simulink library "dspobslib"  (Simulink 6.0)
values from neighbouring files (symbols this model uses):
  D = D + B    [rebuffer_delay.m]
libraries: dspsigattribs x15, simulink x10, dspobslib x3, dspbuff3 x2, dspmtrx3 x2, dspmathops x1
settings Model: RequirementInfo=9  CovMetricSettings=d  Creator=don  LastModifiedBy=mlongfri  ExtModeAutoUpdateStatusClock=off  ProdHWDeviceType=Specified

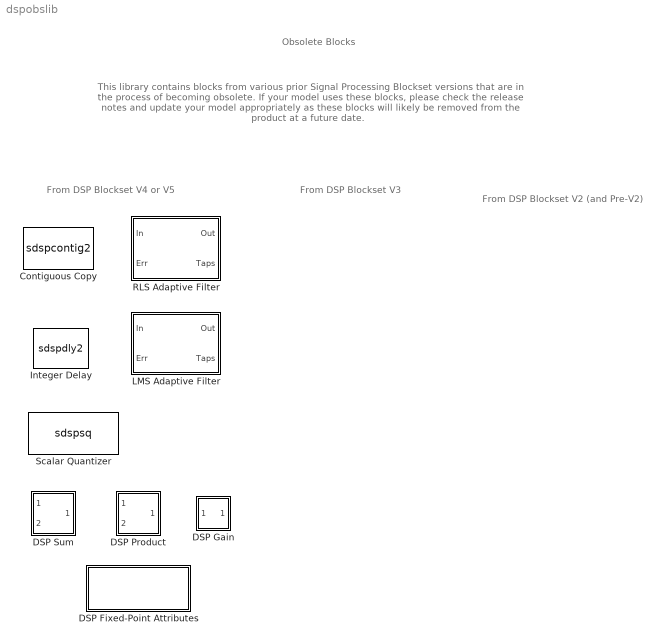
== system dspobslib ==
  note: Obsolete Blocks
  note: This library contains blocks from various prior Signal Processing Blockset versions
      | that are in the process of becoming obsolete. If your model uses these blocks, please
      | check the release notes and update your model appropriately as these blocks will likely
      | be removed from the product at a future date.
  note: From DSP Blockset V4 or V5
  note: From DSP Blockset V3
  note: From DSP Blockset V2
      | (and Pre-V2)
  Contiguous Copy : S-Function  FunctionName=sdspcontig2
      mask Type: Contiguous Copy
      mask Description: Create a contiguous copy of input data.  For use with blocks that only accept contiguous data during simulation or code generation.
      mask Help: web(dspbhelp);
      mask Display: disp('Contiguous\nCopy');
  DSP Fixed-Point Attributes : Subsystem  mask(DSP Fixed-Point Attributes){outputSource=Inherit, outputWordLength=16, outputFracLength=15, accumSource=Inherit, accumWordLength=32, accumFracLength=30, prodOutputSource=Inherit, prodOutputWordLength=32, prodOutputFracLength=30, memorySource=Inherit, memoryWordLength=16, memoryFracLength=15, miscSource=Inherit, roundingMode=Floor, overflowMode=off}
      mask prompts: outputSource "Where from (out)?"; outputWordLength "Word length:"; outputFracLength "Fraction length:"; accumSource "Where from (acc)?"; accumWordLength "Word length:"; accumFracLength "Fraction length:"; prodOutputSource "Where from (po)?"; prodOutputWordLength "Word length:"; prodOutputFracLength "Fraction length:"; memorySource "Where from (mem)?"; memoryWordLength "Word length:"; memoryFracLength "Fraction length:"; miscSource "Where from (misc)?"; roundingMode "Round integer calculations towards:"; overflowMode "Saturate on integer overflow"
      mask help: Sets fixed-point parameters on a model-wide (if at root level) or subsystem-wide basis. Blocks that have 'Inherit from master dialog' will use the parameters specified here unless overridden at a lower level.
      settings: CopyFcn=dspFixptManager('addController');  DeleteFcn=dspFixptManager('removeController');  UndoDeleteFcn=dspFixptManager('addController');  ModelCloseFcn=dspFixptManager('closeModel');  NameChangeFcn=dspFixptManager('changeName');  OpenFcn=dspFixptManager('openUI');
      mask Help: web(dspbhelp);
      mask StyleString: popup(Local|Inherit),edit,edit,popup(Local|Inherit),edit,edit,popup(Local|Inherit),edit,edit,popup(Local|Inherit),edit,edit,popup(Local|Inherit),popup(Floor|Nearest),checkbox
      mask CallbackString: dspblkFPA('out');|||dspblkFPA('acc');|||dspblkFPA('po');|||dspblkFPA('mem');|||dspblkFPA('misc');||
      mask Display: disp('DSP Fixed-Point\nAttributes','horizontalalign','center')
  DSP Gain : Subsystem  mask(DSP Gain){gainValue=1, additionalParams=off, allowOverrides=on, gainMode=Same as input, gainWordLength=16, gainFracLength=15, prodOutputMode=Same as input, prodOutputWordLength=32, prodOutputFracLength=30, roundingMode=Floor, overflowMode=off}
      mask prompts: gainValue "Gain value:"; additionalParams "------- Show additional parameters --------"; allowOverrides "Allow overrides from DSP Fixed-Point Attributes blocks"; gainMode "Fixed-point gain attributes:"; gainWordLength "Gain word length:"; gainFracLength "Gain fraction length:"; prodOutputMode "Fixed-point output attributes:"; prodOutputWordLength "Output word length:"; prodOutputFracLength "Output fraction length:"; roundingMode "Round integer calculations toward:"; overflowMode "Saturate on integer overflow"
      mask help: Apply element-wise gain to input. Any fixed-point settings are ignored for floating-point inputs.
      mask init:
      | iconStr = dspblkdspgain('icon');
      | dspblkdspgain('init');
      mask Help: web(dspbhelp);
      mask StyleString: edit,checkbox,checkbox,popup(Same as input|User-defined),edit,edit,popup(Same as input|User-defined),edit,edit,popup(Floor|Nearest),checkbox
      mask CallbackString: |dspblkdspgain;|dspblkdspgain;|dspblkdspgain;|||dspblkdspgain;|||dspblkdspgain;|dspblkdspgain;
      mask Display:
      | text(0.309,0.5,iconStr,'horizontalalignment','center')
      | plot([0,0],[0,1]);
      | plot([0,1],[0,0.5]);
      | plot([0,1],[1,0.5]);
  DSP Product : Subsystem  mask(DSP Product){allowOverrides=on, prodOutputMode=Same as first input, prodOutputWordLength=32, prodOutputFracLength=30, roundingMode=Floor, overflowMode=off}
      mask prompts: allowOverrides "Allow overrides from DSP Fixed-Point Attributes blocks"; prodOutputMode "Fixed-point output attributes:"; prodOutputWordLength "Output word length:"; prodOutputFracLength "Output fraction length:"; roundingMode "Round integer calculations toward:"; overflowMode "Saturate on integer overflow"
      mask help: Perform element-wise multiplication on two inputs. Any fixed-point settings are ignored for floating-point inputs.
      mask init:
      | dspblksummult('init','Product')
      | dspblksummult('update','Product')
      mask Help: web(dspbhelp);
      mask StyleString: checkbox,popup(Same as first input|User-defined),edit,edit,popup(Floor|Nearest),checkbox
      mask CallbackString: dspblksummult('Product');|dspblksummult('Product');|||dspblksummult('Product');|dspblksummult('Product');
      mask Display:
      | plot((0.5+cos([0:3:360]*pi/180)/3),(0.5+sin([0:3:360]*pi/180)/3))
      | plot([.35,.65],[.35,.65])
      | plot([.65,.35],[.35,.65])
  DSP Sum : Subsystem  mask(DSP Sum){allowOverrides=on, accumMode=Same as first input, accumWordLength=32, accumFracLength=30, roundingMode=Floor, overflowMode=off}
      mask prompts: allowOverrides "Allow overrides from DSP Fixed-Point Attributes blocks"; accumMode "Fixed-point output attributes:"; accumWordLength "Output word length:"; accumFracLength "Output fraction length:"; roundingMode "Round integer calculations toward:"; overflowMode "Saturate on integer overflow"
      mask help: Sum two inputs. Any fixed-point settings are ignored for floating-point inputs.
      mask init:
      | dspblksummult('init','Sum')
      | dspblksummult('update','Sum')
      mask Help: web(dspbhelp);
      mask StyleString: checkbox,popup(Same as first input|User-defined),edit,edit,popup(Floor|Nearest),checkbox
      mask CallbackString: dspblksummult('Sum');|dspblksummult('Sum');|||dspblksummult('Sum');|dspblksummult('Sum');
      mask Display:
      | plot((0.5+cos([0:3:360]*pi/180)/3),(0.5+sin([0:3:360]*pi/180)/3))
      | plot([.5,.5],[.35,.65])
      | plot([.35,.65],[.5,.5])
  Integer Delay : S-Function  FunctionName=sdspdly2  Parameters=delay,ic,reset  mask(Integer Delay){delay=1, ic=0, reset_popup=None}
      mask prompts: delay "Delay (samples):"; ic "Initial conditions:"; reset_popup "Reset port:"
      mask help: Delay discrete-time input by a fixed integer number of sample periods.
      mask init:
      | str = dspblkdly2('icon',&1,delay);
      | dx = 0.01*length(str);
      | reset = reset_popup-1;
      | if (reset == 0)
      | 	s.i1 = 1; s.i1s = '';
      | 	s.i2 = 1; s.i2s = '';
      | else
      | 	s.i1 = 1; s.i1s = 'In';
      | 	s.i2 = 2; s.i2s = 'Rst';
      | end
      mask Help: web(dspbhelp);
      mask StyleString: edit,edit,popup(None|Rising edge|Falling edge|Either edge|Non-zero sample)
      mask Display:
      | text(0.42-dx, 0.4, 'z'); text(0.5-dx, 0.6, str);
      | port_label('input',s.i1,s.i1s);
      | port_label('input',s.i2,s.i2s);
  LMS Adaptive Filter : Subsystem  mask(LMS Adaptive Filter){n=32, mu=.65, ic=0.0, leakage=1.0, normalized=on, Adapt=off, RstPort=None}
      mask prompts: n "FIR filter length:"; mu "Step-size, mu:"; ic "Initial value of filter taps:"; leakage "Leakage factor (0 to 1):"; normalized "Use normalization"; Adapt "Adapt input"; RstPort "Reset input:"
      mask help:
      | Least mean-square (LMS) algorithm for adaptive FIR filtering of input signal.  Energy normalization may optionally be disabled.
      |
      | If 'Adapt input' is checked and the Adapt signal is zero, the algorithm temporarily disables adaptation of the filter coefficients.  A non-zero signal enables filter adaptation.
      |
      | If the 'Reset input' is enabled and the Reset signal transitions appropriately, the filter coefficients are reset to the initial conditions.
      mask init:
      | if normalized, s='nLMS'; else s='LMS'; end
      | dspblkadpt('init');
      mask Help: web(dspbhelp);
      mask StyleString: edit,edit,edit,edit,checkbox,checkbox,popup(None|Rising edge|Falling edge|Either edge|Non-zero sample)
      mask Display: disp(s);
  RLS Adaptive Filter : Subsystem  mask(RLS Adaptive Filter){Ntaps=32, Lambda=1.0, ic=0.0, phi0=0.1, Adapt=off, RstPort=None}
      mask prompts: Ntaps "FIR filter length:"; Lambda "Memory weighting factor (0 to 1):"; ic "Initial value of filter taps:"; phi0 "Initial input variance estimate:"; Adapt "Adapt input"; RstPort "Reset input:"
      mask help:
      | Exponentially weighted recursive least-squares (RLS) algorithm for adaptive FIR filtering of input signal.
      |
      | If 'Adapt input' is checked and the Adapt signal is zero, the algorithm temporarily disables adaptation of the filter coefficients.  A non-zero signal enables filter adaptation.
      |
      | If the 'Reset input' is enabled and the Reset signal transitions appropriately, the filter coefficients are reset to the initial conditions.
      mask init:
      | dspblkadpt('init');
      mask Help: web(dspbhelp);
      mask StyleString: edit,edit,edit,edit,checkbox,popup(None|Rising edge|Falling edge|Either edge|Non-zero sample)
      mask Display: disp('RLS')
  Scalar Quantizer : S-Function  FunctionName=sdspsq  Parameters=Qmode,QparamSource,partitionUnBound,codebook,SearchMethod,tieBreakRule,outQError, invalidin, dtype, idtype, cwdtype,1,1  mask(Scalar Quantizer){Qmode=Encoder, QparamSource=Specify via dialog, partitionUnBound=[   0  1  2  3  4  5    6  7  8    9], codebook=[0.0    1.5     2.5    3.5    4.5   5.5   6.5  7.5  8.5 ], SearchMethod=Binary, tieBreakRule=Choose the lower index, outQError=off, invalidin=Clip and warn, dtype=off, idtype=int32, cwdtype=double}
      mask prompts: Qmode "Quantizer mode:"; QparamSource "Source of quantizer parameters:"; partitionUnBound "Boundary points:"; SearchMethod "Searching method:"; tieBreakRule "Tie-breaking rule:"; outQError "Output the quantization error"; invalidin "Action for out of range input:"; dtype "--------------- Show additional parameters ---------------"; idtype "Output index data type:"; cwdtype "Output data type:"
      mask help:
      | The Scalar Quantizer block has three modes of operation.
      | In Encoder mode, the block maps each input value to a quantization region by comparing the input value to the user-specified quantizer boundary points. The block outputs the index of the associated region.
      | In Decoder mode, the block transforms the input index values into quantized output values, defined by the quantizer codebook.
      | In the Encoder & Decoder mode, the block performs both the encoding and decoding operations. The block outputs the index values and the quantized output values.
      |
      | The Boundary points parameter is a vector of dimension N whose values are arranged in ascending order ([p1 p2 ... pN]). The quantizer codebook is a vector of length (N-1). The quantizer is unbounded if p1 is -inf and pN is inf. When the quantizer is bounded, p1 is the lower bound for the input values. Any input less than p1 is clipped to p1 and then quantized. Similarly, pN is the upper bound for the input values. Any input greater than pN is clipped to pN and is then quantized.
      mask init:
      | [si,so,disp_str]=dspblksq('icon');
      mask Help: web(dspbhelp);
      mask StyleString: popup(Encoder|Decoder|Encoder and decoder),popup(Specify via dialog|Input ports),edit,edit,popup(Linear|Binary),popup(Choose the lower index|Choose the higher index),checkbox,popup(Clip|Clip and warn|Error),checkbox,popup(int8|uint8|int16|uint16|int32|uint32),popup(double|single|int8|uint8|int16|uint16|int32|uint32)
      mask CallbackString: dspblksq|dspblksq||||||dspblksq|dspblksq||
      mask Display:
      | disp(disp_str);
      | port_label('input',si(1).port, si(1).txt);
      | port_label('input',si(2).port, si(2).txt);
      | port_label('input',si(3).port, si(3).txt);
      | port_label('output',so(1).port, so(1).txt);
      | port_label('output',so(2).port, so(2).txt);
      | port_label('output',so(3).port, so(3).txt);

== system dspobslib/DSP Fixed-Point Attributes ==
  Subsystem : Subsystem
      mask Display: disp(' ')

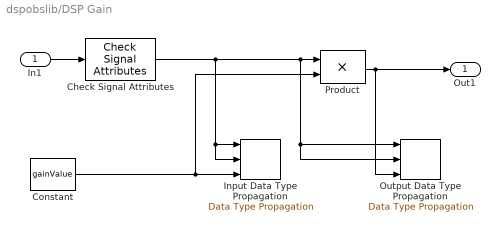
== system dspobslib/DSP Gain ==
  In1 : Inport
  Check Signal Attributes : dspsigattribs/Check Signal Attributes  SigAttribCheckMethod=Matches attributes exactly  Complexity=Ignore  Frame=Ignore  DimsCheckMethod=Ignore  Dimensions=1-D  DatatypeCheckMethod=Is...  DatatypeGeneral=Boolean  DtypeFloatSpecific=Any floating-point  DtypeFixedSpecific=Any fixed-point  DtypeIntSpecific=Any integer  SampleMode=Ignore
  Constant : Constant  Value=gainValue  VectorParams1D=off
  Input Data Type Propagation : simulink/Signal Attributes/Data Type Propagation  PropDataType=sfix(16)  IfRefDouble=double  IfRefSingle=single  IsSigned=IsSigned1 or IsSigned2  NumBitsBase=NumBits1  NumBitsMult=1  NumBitsAdd=0  NumBitsAllowFinal=1:128  PropScaling=2^-10  ValuesUsedBestPrec=[5 -7]  SlopeBase=Slope1  SlopeMult=1  SlopeAdd=0  BiasBase=Bias1  BiasMult=0  BiasAdd=0
  Output Data Type Propagation : simulink/Signal Attributes/Data Type Propagation  PropDataType=sfix(16)  IfRefDouble=double  IfRefSingle=single  IsSigned=IsSigned1 or IsSigned2  NumBitsBase=NumBits1  NumBitsMult=1  NumBitsAdd=0  NumBitsAllowFinal=1:128  PropScaling=2^-10  ValuesUsedBestPrec=[5 -7]  SlopeBase=Slope1  SlopeMult=1  SlopeAdd=0  BiasBase=Bias1  BiasMult=0  BiasAdd=0
  Product : Product
  Out1 : Outport
  wires:
  Check Signal Attributes/1 -> Output Data Type Propagation/2, Output Data Type Propagation/1, Product/1, Input Data Type Propagation/2, Input Data Type Propagation/1
  Constant/1 -> Input Data Type Propagation/3, Product/2
  Product/1 -> Output Data Type Propagation/3, Out1/1
  In1/1 -> Check Signal Attributes/1

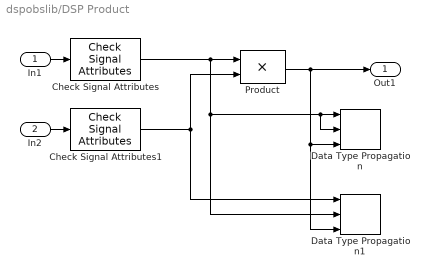
== system dspobslib/DSP Product ==
  In1 : Inport
  In2 : Inport  Port=2
  Check Signal Attributes : dspsigattribs/Check Signal Attributes  SigAttribCheckMethod=Matches attributes exactly  Complexity=Ignore  Frame=Ignore  DimsCheckMethod=Ignore  Dimensions=1-D  DatatypeCheckMethod=Is...  DatatypeGeneral=Boolean  DtypeFloatSpecific=Any floating-point  DtypeFixedSpecific=Any fixed-point  DtypeIntSpecific=Any integer  SampleMode=Ignore
  Check Signal Attributes1 : dspsigattribs/Check Signal Attributes  SigAttribCheckMethod=Matches attributes exactly  Complexity=Ignore  Frame=Ignore  DimsCheckMethod=Ignore  Dimensions=1-D  DatatypeCheckMethod=Is...  DatatypeGeneral=Boolean  DtypeFloatSpecific=Any floating-point  DtypeFixedSpecific=Any fixed-point  DtypeIntSpecific=Any integer  SampleMode=Ignore
  Data Type Propagation : simulink/Signal Attributes/Data Type Propagation  PropDataType=sfix(16)  IfRefDouble=double  IfRefSingle=single  IsSigned=IsSigned1 or IsSigned2  NumBitsBase=NumBits1  NumBitsMult=1  NumBitsAdd=0  NumBitsAllowFinal=1:128  PropScaling=2^-10  ValuesUsedBestPrec=[5 -7]  SlopeBase=Slope1  SlopeMult=1  SlopeAdd=0  BiasBase=Bias1  BiasMult=0  BiasAdd=0
  Data Type Propagation1 : simulink/Signal Attributes/Data Type Propagation  PropDataType=sfix(16)  IfRefDouble=double  IfRefSingle=single  IsSigned=IsSigned1 or IsSigned2  NumBitsBase=NumBits2  NumBitsMult=1  NumBitsAdd=0  NumBitsAllowFinal=1:128  PropScaling=2^-10  ValuesUsedBestPrec=[5 -7]  SlopeBase=Slope2  SlopeMult=1  SlopeAdd=0  BiasBase=Bias2  BiasMult=0  BiasAdd=0
  Product : Product
  Out1 : Outport
  wires:
  Check Signal Attributes1/1 -> Data Type Propagation1/1, Product/2
  Check Signal Attributes/1 -> Data Type Propagation1/2, Data Type Propagation/2, Data Type Propagation/1, Product/1
  Product/1 -> Data Type Propagation1/3, Data Type Propagation/3, Out1/1
  In2/1 -> Check Signal Attributes1/1
  In1/1 -> Check Signal Attributes/1

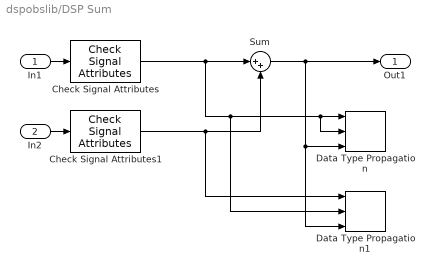
== system dspobslib/DSP Sum ==
  In1 : Inport
  In2 : Inport  Port=2
  Check Signal Attributes : dspsigattribs/Check Signal Attributes  SigAttribCheckMethod=Matches attributes exactly  Complexity=Ignore  Frame=Ignore  DimsCheckMethod=Ignore  Dimensions=1-D  DatatypeCheckMethod=Is...  DatatypeGeneral=Boolean  DtypeFloatSpecific=Any floating-point  DtypeFixedSpecific=Any fixed-point  DtypeIntSpecific=Any integer  SampleMode=Ignore
  Check Signal Attributes1 : dspsigattribs/Check Signal Attributes  SigAttribCheckMethod=Matches attributes exactly  Complexity=Ignore  Frame=Ignore  DimsCheckMethod=Ignore  Dimensions=1-D  DatatypeCheckMethod=Is...  DatatypeGeneral=Boolean  DtypeFloatSpecific=Any floating-point  DtypeFixedSpecific=Any fixed-point  DtypeIntSpecific=Any integer  SampleMode=Ignore
  Data Type Propagation : simulink/Signal Attributes/Data Type Propagation  PropDataType=sfix(16)  IfRefDouble=double  IfRefSingle=single  IsSigned=IsSigned1 or IsSigned2  NumBitsBase=NumBits1  NumBitsMult=1  NumBitsAdd=0  NumBitsAllowFinal=1:128  PropScaling=2^-10  ValuesUsedBestPrec=[5 -7]  SlopeBase=Slope1  SlopeMult=1  SlopeAdd=0  BiasBase=Bias1  BiasMult=0  BiasAdd=0
  Data Type Propagation1 : simulink/Signal Attributes/Data Type Propagation  PropDataType=sfix(16)  IfRefDouble=double  IfRefSingle=single  IsSigned=IsSigned1 or IsSigned2  NumBitsBase=NumBits2  NumBitsMult=1  NumBitsAdd=0  NumBitsAllowFinal=1:128  PropScaling=2^-10  ValuesUsedBestPrec=[5 -7]  SlopeBase=Slope2  SlopeMult=1  SlopeAdd=0  BiasBase=Bias2  BiasMult=0  BiasAdd=0
  Sum : Sum  Inputs=|++
  Out1 : Outport
  wires:
  Check Signal Attributes1/1 -> Data Type Propagation1/1, Sum/2
  Check Signal Attributes/1 -> Data Type Propagation1/2, Data Type Propagation/2, Data Type Propagation/1, Sum/1
  In2/1 -> Check Signal Attributes1/1
  Sum/1 -> Data Type Propagation1/3, Data Type Propagation/3, Out1/1
  In1/1 -> Check Signal Attributes/1

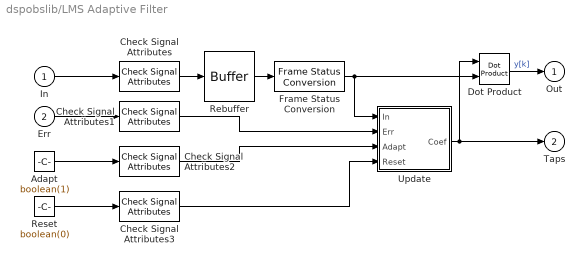
== system dspobslib/LMS Adaptive Filter ==
  In : Inport
  Err : Inport  Port=2
  Adapt : Constant  Value=boolean(1)
  Check Signal Attributes{,1..3} (4 alike) : dspsigattribs/Check Signal Attributes  SigAttribCheckMethod=Does not match attributes exactly  Complexity=Ignore  Frame=Sample-based  DimsCheckMethod=Is...  Dimensions=Scalar (1-D or 2-D)  DatatypeCheckMethod=Ignore  DatatypeGeneral=Boolean  DtypeFloatSpecific=Any floating-point  DtypeFixedSpecific=Any fixed-point  DtypeIntSpecific=Any integer  SampleMode=Ignore
  Dot Product : simulink/Math Operations/Dot Product
  Frame Status Conversion : dspsigattribs/Frame Status Conversion  growRefPort=off  outframe=Sample-based
  Rebuffer : dspbuff3/Buffer  N=n  V=n-1  ic=0
  Reset : Constant  Value=boolean(0)
  Update : Subsystem
  Out : Outport  InitialOutput=0
  Taps : Outport  Port=2  InitialOutput=0
  wires:
  Dot Product/1 -> Out/1  "y[k]"
  Update/1(Coef) -> Taps/1, Dot Product/1
  Rebuffer/1 -> Frame Status Conversion/1
  In/1 -> Check Signal Attributes/1
  Check Signal Attributes/1 -> Rebuffer/1
  Err/1 -> Check Signal Attributes1/1
  Check Signal Attributes1/1 -> Update/2(Err)
  Adapt/1 -> Check Signal Attributes2/1
  Check Signal Attributes2/1 -> Update/3(Adapt)
  Frame Status Conversion/1 -> Update/1(In), Dot Product/2
  Reset/1 -> Check Signal Attributes3/1
  Check Signal Attributes3/1 -> Update/4(Reset)

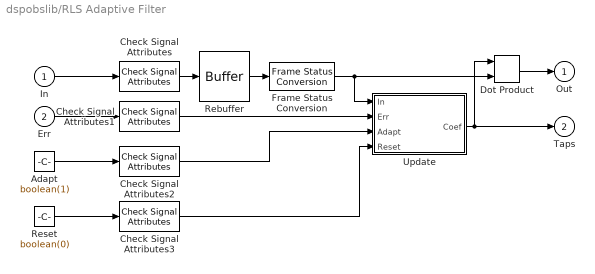
== system dspobslib/RLS Adaptive Filter ==
  In : Inport
  Err : Inport  Port=2
  Adapt : Constant  Value=boolean(1)
  Check Signal Attributes{,1..3} (4 alike) : dspsigattribs/Check Signal Attributes  SigAttribCheckMethod=Does not match attributes exactly  Complexity=Ignore  Frame=Sample-based  DimsCheckMethod=Is...  Dimensions=Scalar (1-D or 2-D)  DatatypeCheckMethod=Ignore  DatatypeGeneral=Boolean  DtypeFloatSpecific=Any floating-point  DtypeFixedSpecific=Any fixed-point  DtypeIntSpecific=Any integer  SampleMode=Ignore
  Dot Product : simulink/Math Operations/Dot Product
  Frame Status Conversion : dspsigattribs/Frame Status Conversion  growRefPort=off  outframe=Sample-based
  Rebuffer : dspbuff3/Buffer  N=Ntaps  V=Ntaps-1  ic=0
  Reset : Constant  Value=boolean(0)
  Update : Subsystem
  Out : Outport  InitialOutput=0
  Taps : Outport  Port=2  InitialOutput=0
  wires:
  Dot Product/1 -> Out/1
  Update/1(Coef) -> Taps/1, Dot Product/1
  Rebuffer/1 -> Frame Status Conversion/1
  In/1 -> Check Signal Attributes/1
  Check Signal Attributes/1 -> Rebuffer/1
  Err/1 -> Check Signal Attributes1/1
  Check Signal Attributes1/1 -> Update/2(Err)
  Adapt/1 -> Check Signal Attributes2/1
  Check Signal Attributes2/1 -> Update/3(Adapt)
  Frame Status Conversion/1 -> Update/1(In), Dot Product/2
  Reset/1 -> Check Signal Attributes3/1
  Check Signal Attributes3/1 -> Update/4(Reset)

== system dspobslib/DSP Fixed-Point Attributes/Subsystem ==

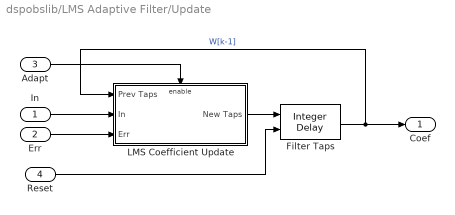
== system dspobslib/LMS Adaptive Filter/Update ==
  In : Inport
  Err : Inport  Port=2
  Adapt : Inport  Port=3
  Reset : Inport  Port=4
  Filter Taps : dspobslib/Integer Delay  delay=1  ic=ic  reset_popup=Non-zero sample
  LMS Coefficient Update : Subsystem  TreatAsAtomicUnit=on
  Coef : Outport  InitialOutput=0
  wires:
  LMS Coefficient Update/1(New Taps) -> Filter Taps/1
  Err/1 -> LMS Coefficient Update/3(Err)
  In/1 -> LMS Coefficient Update/2(In)
  Filter Taps/1 -> Coef/1, LMS Coefficient Update/1(Prev Taps)  "W[k-1]"
  Adapt/1 -> LMS Coefficient Update/Enable
  Reset/1 -> Filter Taps/2

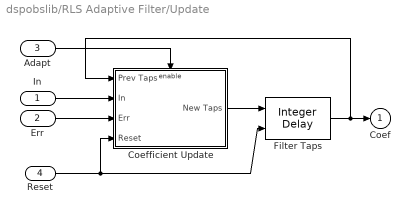
== system dspobslib/RLS Adaptive Filter/Update ==
  In : Inport
  Err : Inport  Port=2
  Adapt : Inport  Port=3
  Reset : Inport  Port=4
  Coefficient Update : Subsystem  TreatAsAtomicUnit=on
  Filter Taps : dspobslib/Integer Delay  delay=1  ic=ic  reset_popup=Non-zero sample
  Coef : Outport  InitialOutput=0
  wires:
  Err/1 -> Coefficient Update/3(Err)
  Filter Taps/1 -> Coef/1, Coefficient Update/1(Prev Taps)
  Coefficient Update/1(New Taps) -> Filter Taps/1
  In/1 -> Coefficient Update/2(In)
  Adapt/1 -> Coefficient Update/Enable
  Reset/1 -> Filter Taps/2, Coefficient Update/4(Reset)

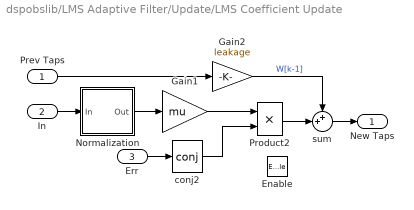
== system dspobslib/LMS Adaptive Filter/Update/LMS Coefficient Update ==
  Prev Taps : Inport
  In : Inport  Port=2
  Err : Inport  Port=3
  Enable : EnablePort  ZeroCross=off
  Gain1 : Gain  Gain=mu  SaturateOnIntegerOverflow=on
  Gain2 : Gain  Gain=leakage  SaturateOnIntegerOverflow=on
  Normalization : Subsystem  mask(Replaceable Contents){oname=Normalization, osrc=dspmathops/Normalization, oargs={'NormType','Squared 2-norm','Bias','1e-10'}, replace=~normalized}
      mask prompts: oname "Relative name of blocks to replace:"; osrc "Simulink path to each source block:"; oargs "Parameter/value pairs to each block:"; replace "Replace with short-circuit:"
      mask help: Configurable subsystem holding blocks which may be replaced by virtual short-circuits (muxes) when not needed.
      mask init:
      | opts.name = oname; opts.src = osrc; opts.args = oargs;
      | dspskipblk(gcb,opts,replace);
  Product2 : Product  SaturateOnIntegerOverflow=on  InputSameDT=on
  conj2 : Math  Operator=conj  SaturateOnIntegerOverflow=on
  sum : Sum  Inputs=++|  SaturateOnIntegerOverflow=on  InputSameDT=on
  New Taps : Outport  InitialOutput=ic
  wires:
  conj2/1 -> Product2/2
  Gain1/1 -> Product2/1
  Normalization/1(Out) -> Gain1/1
  Product2/1 -> sum/2
  Gain2/1 -> sum/1  "W[k-1]"
  Prev Taps/1 -> Gain2/1
  In/1 -> Normalization/1(In)
  sum/1 -> New Taps/1
  Err/1 -> conj2/1

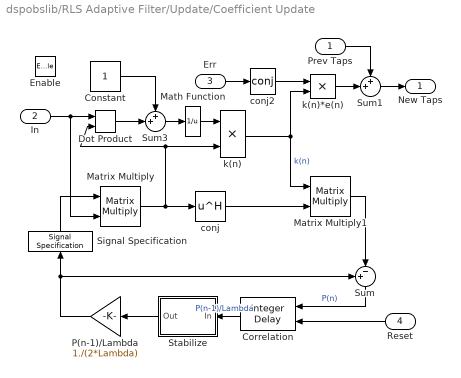
== system dspobslib/RLS Adaptive Filter/Update/Coefficient Update ==
  Prev Taps : Inport
  In : Inport  Port=2
  Err : Inport  Port=3
  Reset : Inport  Orientation=left  Port=4
  Enable : EnablePort  ZeroCross=off
  Constant : Constant
  Correlation : dspobslib/Integer Delay  Orientation=left  delay=1  ic=eye(Ntaps)./phi0  reset_popup=Either edge
  Dot Product : simulink/Math Operations/Dot Product
  Math Function : Math  Operator=reciprocal  SaturateOnIntegerOverflow=on
  Matrix Multiply : dspmtrx3/Matrix Multiply  numInputPorts=2  OptimizationLevel=None
  Matrix Multiply1 : dspmtrx3/Matrix Multiply  numInputPorts=2  OptimizationLevel=None
  P(n-1)/Lambda : Gain  Orientation=left  Gain=1./(2*Lambda)  SaturateOnIntegerOverflow=on
  Signal Specification : simulink/Signal Attributes/Signal Specification  Orientation=up  D=[Ntaps Ntaps]  Ts=-1  DataType=auto  OutDataType=sfix(16)  OutScaling=2^0
      settings: SignalType=auto  SamplingMode=auto
  Stabilize : Subsystem  Orientation=left
  Sum : Sum  Orientation=down  Inputs=+-|  SaturateOnIntegerOverflow=on  InputSameDT=on
  Sum1 : Sum  Inputs=++|  SaturateOnIntegerOverflow=on  InputSameDT=on
  Sum3 : Sum  Inputs=++|  SaturateOnIntegerOverflow=on  InputSameDT=on
  conj : Math  Operator=hermitian  SaturateOnIntegerOverflow=on
  conj2 : Math  Operator=conj  SaturateOnIntegerOverflow=on
  k(n) : Product  SaturateOnIntegerOverflow=on  InputSameDT=on
  k(n)*e(n) : Product  SaturateOnIntegerOverflow=on  InputSameDT=on
  New Taps : Outport  InitialOutput=ic
  wires:
  k(n)*e(n)/1 -> Sum1/2
  Constant/1 -> Sum3/1
  Dot Product/1 -> Sum3/2
  In/1 -> Dot Product/1, Matrix Multiply/2
  Sum3/1 -> Math Function/1
  Matrix Multiply/1 -> Dot Product/2, k(n)/2, conj/1
  conj/1 -> Matrix Multiply1/2
  Matrix Multiply1/1 -> Sum/2
  Sum/1 -> Correlation/1  "P(n)"
  k(n)/1 -> Matrix Multiply1/1, k(n)*e(n)/2  "k(n)"
  conj2/1 -> k(n)*e(n)/1
  Prev Taps/1 -> Sum1/1
  Err/1 -> conj2/1
  Sum1/1 -> New Taps/1
  Stabilize/1(Out) -> P(n-1)/Lambda/1
  P(n-1)/Lambda/1 -> Sum/1, Signal Specification/1
  Signal Specification/1 -> Matrix Multiply/1
  Math Function/1 -> k(n)/1
  Correlation/1 -> Stabilize/1(In)  "P(n-1)/Lambda"
  Reset/1 -> Correlation/2

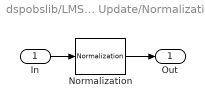
== system dspobslib/LMS Adaptive Filter/Update/LMS Coefficient Update/Normalization ==
  In : Inport
  Normalization : dspmathops/Normalization  NormType=Squared 2-norm  Bias=1e-10
  Out : Outport  InitialOutput=0
  wires:
  In/1 -> Normalization/1
  Normalization/1 -> Out/1

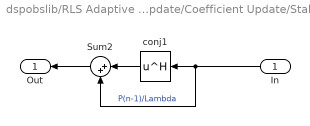
== system dspobslib/RLS Adaptive Filter/Update/Coefficient Update/Stabilize ==
  In : Inport  Orientation=left
  Sum2 : Sum  Orientation=left  Inputs=|++  SaturateOnIntegerOverflow=on  InputSameDT=on
  conj1 : Math  Orientation=left  Operator=hermitian  SaturateOnIntegerOverflow=on
  Out : Outport  Orientation=left
  wires:
  In/1 -> conj1/1, Sum2/2  "P(n-1)/Lambda"
  conj1/1 -> Sum2/1
  Sum2/1 -> Out/1
